simulink model "adc_16g_asnt"  (R2018a)
settings: Solver=VariableStepAuto  StartTime=0.0  StopTime=10.0  RelTol=1e-3
libraries: xbsIndex_r4 x18
settings Model: Creator=jkocz  LastModifiedBy=wei
settings CodeAppCC: StateflowObjectComments=on

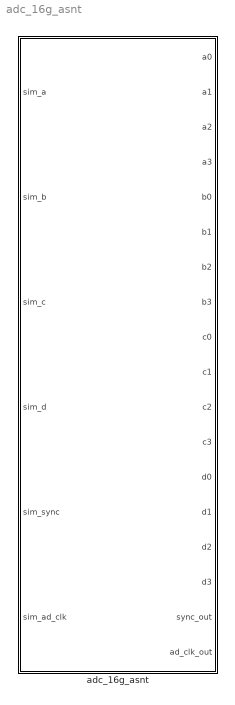
== system adc_16g_asnt ==
  adc_16g_asnt : Subsystem  Tag=xps:adc_4x16g_asnt  AncestorBlock=xps_adc/ADCs/adc_5g_e2v  mask(E2V_5g_adc){}
      mask init:
      | adc_16g_asnt_init(gcb);

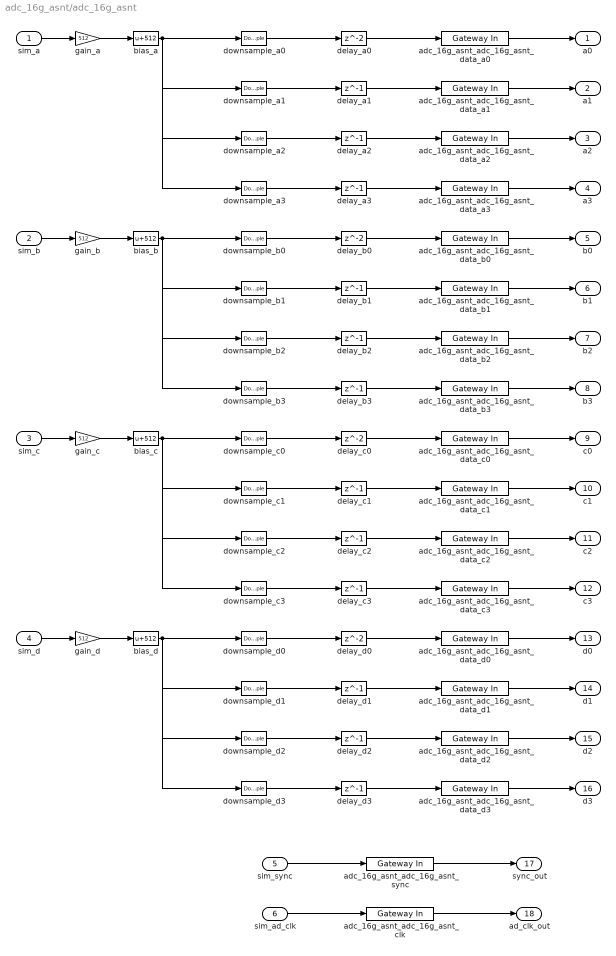
== system adc_16g_asnt/adc_16g_asnt ==
  sim_a : Inport
  sim_b : Inport  Port=2
  sim_c : Inport  Port=3
  sim_d : Inport  Port=4
  sim_sync : Inport  Port=5
  sim_ad_clk : Inport  Port=6
  adc_16g_asnt_adc_16g_asnt_clk : xbsIndex_r4/Gateway In  gui_display_data_type=Fixed-point  arith_type=Boolean  n_bits=16  bin_pt=14  preci_type=Single  exp_width=8  frac_width=24  rows=1  columns=1  quantization="Round  (unbiased: +/- Inf)"  overflow=Saturate  period=1  UseAsADC=off  ADCChannel='1'  interface=None  automatic_assignment=on  address_offset=hex2dec('00')  intf_name=''  intf_description=''  default_value=0  timing_constraint=None  locs_specified=off  LOCs={}  io_standard={}  inherit_from_input=off  hdl_port=on  dbl_ovrd=off  block_type=gatewayin
  adc_16g_asnt_adc_16g_asnt_data_a{0..3} (4 alike) : xbsIndex_r4/Gateway In  gui_display_data_type=Fixed-point  arith_type=Unsigned  n_bits=4  bin_pt=0  preci_type=Single  exp_width=8  frac_width=24  rows=1  columns=1  quantization=Truncate  overflow=Wrap  period=1  UseAsADC=off  ADCChannel='1'  interface=None  automatic_assignment=on  address_offset=hex2dec('00')  intf_name=''  intf_description=''  default_value=0  timing_constraint=None  locs_specified=off  LOCs={}  io_standard={}  inherit_from_input=off  hdl_port=on  dbl_ovrd=off  block_type=gatewayin
  adc_16g_asnt_adc_16g_asnt_data_b{0..3} (4 alike) : xbsIndex_r4/Gateway In  gui_display_data_type=Fixed-point  arith_type=Unsigned  n_bits=4  bin_pt=0  preci_type=Single  exp_width=8  frac_width=24  rows=1  columns=1  quantization=Truncate  overflow=Wrap  period=1  UseAsADC=off  ADCChannel='1'  interface=None  automatic_assignment=on  address_offset=hex2dec('00')  intf_name=''  intf_description=''  default_value=0  timing_constraint=None  locs_specified=off  LOCs={}  io_standard={}  inherit_from_input=off  hdl_port=on  dbl_ovrd=off  block_type=gatewayin
  adc_16g_asnt_adc_16g_asnt_data_c{0..3} (4 alike) : xbsIndex_r4/Gateway In  gui_display_data_type=Fixed-point  arith_type=Unsigned  n_bits=4  bin_pt=0  preci_type=Single  exp_width=8  frac_width=24  rows=1  columns=1  quantization=Truncate  overflow=Wrap  period=1  UseAsADC=off  ADCChannel='1'  interface=None  automatic_assignment=on  address_offset=hex2dec('00')  intf_name=''  intf_description=''  default_value=0  timing_constraint=None  locs_specified=off  LOCs={}  io_standard={}  inherit_from_input=off  hdl_port=on  dbl_ovrd=off  block_type=gatewayin
  adc_16g_asnt_adc_16g_asnt_data_d{0..3} (4 alike) : xbsIndex_r4/Gateway In  gui_display_data_type=Fixed-point  arith_type=Unsigned  n_bits=4  bin_pt=0  preci_type=Single  exp_width=8  frac_width=24  rows=1  columns=1  quantization=Truncate  overflow=Wrap  period=1  UseAsADC=off  ADCChannel='1'  interface=None  automatic_assignment=on  address_offset=hex2dec('00')  intf_name=''  intf_description=''  default_value=0  timing_constraint=None  locs_specified=off  LOCs={}  io_standard={}  inherit_from_input=off  hdl_port=on  dbl_ovrd=off  block_type=gatewayin
  adc_16g_asnt_adc_16g_asnt_sync : xbsIndex_r4/Gateway In  gui_display_data_type=Fixed-point  arith_type=Boolean  n_bits=16  bin_pt=14  preci_type=Single  exp_width=8  frac_width=24  rows=1  columns=1  quantization="Round  (unbiased: +/- Inf)"  overflow=Saturate  period=1  UseAsADC=off  ADCChannel='1'  interface=None  automatic_assignment=on  address_offset=hex2dec('00')  intf_name=''  intf_description=''  default_value=0  timing_constraint=None  locs_specified=off  LOCs={}  io_standard={}  inherit_from_input=off  hdl_port=on  dbl_ovrd=off  block_type=gatewayin
  bias_a : Bias  Bias=512  SaturateOnIntegerOverflow=on
  bias_b : Bias  Bias=512  SaturateOnIntegerOverflow=on
  bias_c : Bias  Bias=512  SaturateOnIntegerOverflow=on
  bias_d : Bias  Bias=512  SaturateOnIntegerOverflow=on
  delay_a0 : Delay  InitialCondition=0  InputProcessing=Inherited
  delay_a1 : Delay  DelayLength=1  InitialCondition=0  InputProcessing=Inherited
  delay_a2 : Delay  DelayLength=1  InitialCondition=0  InputProcessing=Inherited
  delay_a3 : Delay  DelayLength=1  InitialCondition=0  InputProcessing=Inherited
  delay_b0 : Delay  InitialCondition=0  InputProcessing=Inherited
  delay_b1 : Delay  DelayLength=1  InitialCondition=0  InputProcessing=Inherited
  delay_b2 : Delay  DelayLength=1  InitialCondition=0  InputProcessing=Inherited
  delay_b3 : Delay  DelayLength=1  InitialCondition=0  InputProcessing=Inherited
  delay_c0 : Delay  InitialCondition=0  InputProcessing=Inherited
  delay_c1 : Delay  DelayLength=1  InitialCondition=0  InputProcessing=Inherited
  delay_c2 : Delay  DelayLength=1  InitialCondition=0  InputProcessing=Inherited
  delay_c3 : Delay  DelayLength=1  InitialCondition=0  InputProcessing=Inherited
  delay_d0 : Delay  InitialCondition=0  InputProcessing=Inherited
  delay_d1 : Delay  DelayLength=1  InitialCondition=0  InputProcessing=Inherited
  delay_d2 : Delay  DelayLength=1  InitialCondition=0  InputProcessing=Inherited
  delay_d3 : Delay  DelayLength=1  InitialCondition=0  InputProcessing=Inherited
  downsample_a0 : DownSample  N=4  RateOptions=Allow multirate processing
  downsample_a1 : DownSample  N=4  phase=1  RateOptions=Allow multirate processing
  downsample_a2 : DownSample  N=4  phase=2  RateOptions=Allow multirate processing
  downsample_a3 : DownSample  N=4  phase=3  RateOptions=Allow multirate processing
  downsample_b0 : DownSample  N=4  RateOptions=Allow multirate processing
  downsample_b1 : DownSample  N=4  phase=1  RateOptions=Allow multirate processing
  downsample_b2 : DownSample  N=4  phase=2  RateOptions=Allow multirate processing
  downsample_b3 : DownSample  N=4  phase=3  RateOptions=Allow multirate processing
  downsample_c0 : DownSample  N=4  RateOptions=Allow multirate processing
  downsample_c1 : DownSample  N=4  phase=1  RateOptions=Allow multirate processing
  downsample_c2 : DownSample  N=4  phase=2  RateOptions=Allow multirate processing
  downsample_c3 : DownSample  N=4  phase=3  RateOptions=Allow multirate processing
  downsample_d0 : DownSample  N=4  RateOptions=Allow multirate processing
  downsample_d1 : DownSample  N=4  phase=1  RateOptions=Allow multirate processing
  downsample_d2 : DownSample  N=4  phase=2  RateOptions=Allow multirate processing
  downsample_d3 : DownSample  N=4  phase=3  RateOptions=Allow multirate processing
  gain_a : Gain  Gain=512  SaturateOnIntegerOverflow=on  OutDataTypeStr=Inherit: Same as input  ParamDataTypeStr=Inherit: Same as input
  gain_b : Gain  Gain=512  SaturateOnIntegerOverflow=on  OutDataTypeStr=Inherit: Same as input  ParamDataTypeStr=Inherit: Same as input
  gain_c : Gain  Gain=512  SaturateOnIntegerOverflow=on  OutDataTypeStr=Inherit: Same as input  ParamDataTypeStr=Inherit: Same as input
  gain_d : Gain  Gain=512  SaturateOnIntegerOverflow=on  OutDataTypeStr=Inherit: Same as input  ParamDataTypeStr=Inherit: Same as input
  a0 : Outport
  a1 : Outport  Port=2
  a2 : Outport  Port=3
  a3 : Outport  Port=4
  b0 : Outport  Port=5
  b1 : Outport  Port=6
  b2 : Outport  Port=7
  b3 : Outport  Port=8
  c0 : Outport  Port=9
  c1 : Outport  Port=10
  c2 : Outport  Port=11
  c3 : Outport  Port=12
  d0 : Outport  Port=13
  d1 : Outport  Port=14
  d2 : Outport  Port=15
  d3 : Outport  Port=16
  sync_out : Outport  Port=17
  ad_clk_out : Outport  Port=18
  wires:
  adc_16g_asnt_adc_16g_asnt_clk/1 -> ad_clk_out/1
  sim_ad_clk/1 -> adc_16g_asnt_adc_16g_asnt_clk/1
  adc_16g_asnt_adc_16g_asnt_sync/1 -> sync_out/1
  sim_sync/1 -> adc_16g_asnt_adc_16g_asnt_sync/1
  adc_16g_asnt_adc_16g_asnt_data_d3/1 -> d3/1
  delay_d3/1 -> adc_16g_asnt_adc_16g_asnt_data_d3/1
  downsample_d3/1 -> delay_d3/1
  adc_16g_asnt_adc_16g_asnt_data_d2/1 -> d2/1
  delay_d2/1 -> adc_16g_asnt_adc_16g_asnt_data_d2/1
  downsample_d2/1 -> delay_d2/1
  adc_16g_asnt_adc_16g_asnt_data_d1/1 -> d1/1
  delay_d1/1 -> adc_16g_asnt_adc_16g_asnt_data_d1/1
  downsample_d1/1 -> delay_d1/1
  adc_16g_asnt_adc_16g_asnt_data_d0/1 -> d0/1
  delay_d0/1 -> adc_16g_asnt_adc_16g_asnt_data_d0/1
  downsample_d0/1 -> delay_d0/1
  bias_d/1 -> downsample_d3/1, downsample_d2/1, downsample_d1/1, downsample_d0/1
  gain_d/1 -> bias_d/1
  sim_d/1 -> gain_d/1
  adc_16g_asnt_adc_16g_asnt_data_c3/1 -> c3/1
  delay_c3/1 -> adc_16g_asnt_adc_16g_asnt_data_c3/1
  downsample_c3/1 -> delay_c3/1
  adc_16g_asnt_adc_16g_asnt_data_c2/1 -> c2/1
  delay_c2/1 -> adc_16g_asnt_adc_16g_asnt_data_c2/1
  downsample_c2/1 -> delay_c2/1
  adc_16g_asnt_adc_16g_asnt_data_c1/1 -> c1/1
  delay_c1/1 -> adc_16g_asnt_adc_16g_asnt_data_c1/1
  downsample_c1/1 -> delay_c1/1
  adc_16g_asnt_adc_16g_asnt_data_c0/1 -> c0/1
  delay_c0/1 -> adc_16g_asnt_adc_16g_asnt_data_c0/1
  downsample_c0/1 -> delay_c0/1
  bias_c/1 -> downsample_c3/1, downsample_c2/1, downsample_c1/1, downsample_c0/1
  gain_c/1 -> bias_c/1
  sim_c/1 -> gain_c/1
  adc_16g_asnt_adc_16g_asnt_data_b3/1 -> b3/1
  delay_b3/1 -> adc_16g_asnt_adc_16g_asnt_data_b3/1
  downsample_b3/1 -> delay_b3/1
  adc_16g_asnt_adc_16g_asnt_data_b2/1 -> b2/1
  delay_b2/1 -> adc_16g_asnt_adc_16g_asnt_data_b2/1
  downsample_b2/1 -> delay_b2/1
  adc_16g_asnt_adc_16g_asnt_data_b1/1 -> b1/1
  delay_b1/1 -> adc_16g_asnt_adc_16g_asnt_data_b1/1
  downsample_b1/1 -> delay_b1/1
  adc_16g_asnt_adc_16g_asnt_data_b0/1 -> b0/1
  delay_b0/1 -> adc_16g_asnt_adc_16g_asnt_data_b0/1
  downsample_b0/1 -> delay_b0/1
  bias_b/1 -> downsample_b3/1, downsample_b2/1, downsample_b1/1, downsample_b0/1
  gain_b/1 -> bias_b/1
  sim_b/1 -> gain_b/1
  adc_16g_asnt_adc_16g_asnt_data_a3/1 -> a3/1
  delay_a3/1 -> adc_16g_asnt_adc_16g_asnt_data_a3/1
  downsample_a3/1 -> delay_a3/1
  adc_16g_asnt_adc_16g_asnt_data_a2/1 -> a2/1
  delay_a2/1 -> adc_16g_asnt_adc_16g_asnt_data_a2/1
  downsample_a2/1 -> delay_a2/1
  adc_16g_asnt_adc_16g_asnt_data_a1/1 -> a1/1
  delay_a1/1 -> adc_16g_asnt_adc_16g_asnt_data_a1/1
  downsample_a1/1 -> delay_a1/1
  adc_16g_asnt_adc_16g_asnt_data_a0/1 -> a0/1
  delay_a0/1 -> adc_16g_asnt_adc_16g_asnt_data_a0/1
  downsample_a0/1 -> delay_a0/1
  bias_a/1 -> downsample_a3/1, downsample_a2/1, downsample_a1/1, downsample_a0/1
  gain_a/1 -> bias_a/1
  sim_a/1 -> gain_a/1
